simulink model "ALL_JP360_DBW_V6_5_1103"  (R2022a)
settings: Solver=FixedStepAuto  StartTime=0.0  StopTime=inf  FixedStep=0.01  RelTol=1e-3  EnableMultiTasking=on
model workspace (MAT data in the model file):
  g = 9.8
undefined symbols (not defined in the file or in its folder): canChannel, delta_v_p, IPM_Line_C0, IPM_Line_C1, IPM_Line_C2, IPM_Line_C3, M, M_p, MRR_ObjDistX, MRR_ObjDistY, MRR_ObjFusionCamID, MRR_ObjFusionSig, MRR_ObjID, MRR_ObjRelVelX, MRR_ObjRelVelY, MRR_ObjType, MRR_ObjUpdFlg, none, obj_vaild, untracktime, V, videoinput
libraries: canfdmsglib x230, canfdlib x76, slpidlib x24, simulink x18, dspstat3 x14, ctrlSharedLib x1, simulink_extras x1, imaqlib x1, realtime_pacer_lib x1, dspvision x1, visionsinks x1
(part 4 of 55)

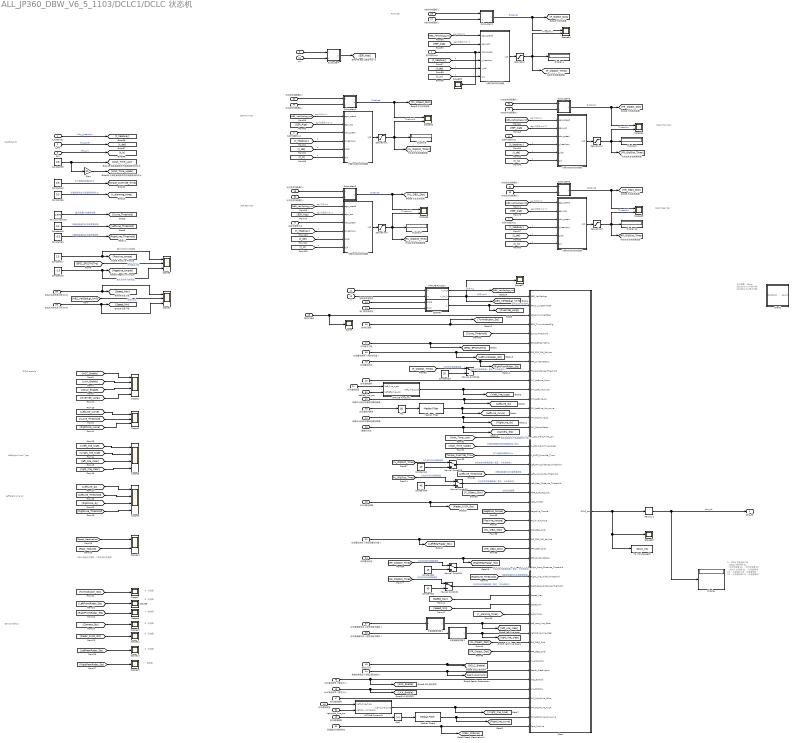
== system ALL_JP360_DBW_V6_5_1103/DCLC1/DCLC状态机 ==
  note: Coefficients
  note: 1表示未越过车道线，2表示越过车道线
  note: 0：无故障
  note: Front Car
  note: Left/Right Line Type
  note: DCLC enable
  note: 运行周期：10ms
      | condition为1开始计数；
      | condition为0停止计数；
  note: ego加速度m/s^2
  note: s
  note: s
  note: s
  note: ego加速度m/s^2
  note: s
  note: 0	：DCLC功能关闭
      | 10	：DCLC功能受限
      | 11	：允许左变道
      | 12	：允许右变道
      | 13	：允许左/右变道
      | 21	：左变道等待
      | 22	：左变道中
      | 23	：左变道回退
      | 24	：左变道结束
      | 31	：右变道等待
      | 32	：右变道中
      | 33	：右变道回退
      | 34	：右变道结束
  note: ego车速m/s
  note: s
  note: s
  note: s
  note: s
  note: ego车速m/s
  note: s
  note: s
  note: ego加速度m/s^2
  note: ego车速m/s
  note: s
  note: ego加速度m/s^2
  note: ego车速m/s
  note: s
  note: s
  note: ego车速m/s
  note: ego加速度m/s^2
  note: s
  note: s
  note: Left/Right Line dy
  note: Left Front Car
  note: Right Front Car
  note: Right Rear Car
  note: Left Rear Car
  note: 0：无故障
  note: 7：有故障
  note: 0：无故障
  note: 0：无故障
  note: 0：无故障
  note: 7：有故障
  note: Sensor Status
  t_headway : Inport
  t_del : Inport  Port=2
  t_lc : Inport  Port=3
  前车速度m/s : Inport  Port=4
  左前车速度m/s : Inport  Port=5
  右前车速度m/s : Inport  Port=6
  右后车速度m/s : Inport  Port=7
  左后车速度m/s : Inport  Port=8
  ax : Inport  Port=9
  ay : Inport  Port=10
  vx : Inport  Port=11
  vy : Inport  Port=12
  刹车信号有效性 : Inport  Port=13
  油门信号有效性 : Inport  Port=14
  转向灯请求 : Inport  Port=15
  转向灯故障 : Inport  Port=16
  方向盘手力矩 : Inport  Port=17
  左前雷达故障（用右前代替） : Inport  Port=18
  右前雷达状态 : Inport  Port=19
  左车道线颜色 : Inport  Port=20
  左车道线类型 : Inport  Port=21
  后轴中心到左车道线的横向距离 : Inport  Port=22
  左车道线的曲率 : Inport  Port=23
  后轴中心到右车道线的横向距离 : Inport  Port=24
  摄像头状态 : Inport  Port=25
  与前车的距离的x : Inport  Port=26
  与前车的距离的y : Inport  Port=27
  1V1R雷达故障 : Inport  Port=28
  与左后车的距离的x : Inport  Port=29
  与左后车的距离的y : Inport  Port=30
  左后雷达失效（用右后雷达代替） : Inport  Port=31
  与右后车的距离的x : Inport  Port=32
  与右后车的距离的y : Inport  Port=33
  右后雷达状态 : Inport  Port=34
  DCLC失效车速上限/km/h : Inport  Port=35
  DCLC失效车速下限/km/h : Inport  Port=36
  左车道清晰状态（信号名暂不确定） : Inport  Port=37
  右车道清晰状态（信号名暂不确定） : Inport  Port=38
  与左前车的距离的x : Inport  Port=39
  与左前车的距离的y : Inport  Port=40
  与右前车的距离的x : Inport  Port=41
  与右前车的距离的y : Inport  Port=42
  DCLC开关 : Inport  Port=43
  换道结束标志（DCLC算法给出） : Inport  Port=44
  ACC激活信号（暂定为1） : Inport  Port=45
  LKA激活信号（暂定为1） : Inport  Port=46
  右车道线颜色 : Inport  Port=47
  右车道线类型 : Inport  Port=48
  右车道线曲率 : Inport  Port=49
  变道越过车道线标志 : Inport  Port=50
  leftleft_line_pro : Inport  Port=51
  rightright_line_pro : Inport  Port=52
  Abs : Abs  SaturateOnIntegerOverflow=off
  Abs1 : Abs  SaturateOnIntegerOverflow=off
  Chart : Stateflow chart  TreatAsAtomicUnit=on
  Chart1 : Stateflow chart  TreatAsAtomicUnit=on
  Constant16 : Constant  Value=-1.5  OutDataTypeStr=single
  Constant17 : Constant  Value=1.5  OutDataTypeStr=single
  Constant23 : Constant  Value=20  OutDataTypeStr=single
  Constant38 : Constant  Value=0.5  OutDataTypeStr=single
  Constant40 : Constant  Value=0.5
  Constant{44,46,60,62} (4 alike) : Constant  Value=45  OutDataTypeStr=single
  Constant45 : Constant  Value=0.5  OutDataTypeStr=single
  Constant61 : Constant  Value=-0.5  OutDataTypeStr=single
  Constant66 : Constant  Value=0.5  OutDataTypeStr=single
  Display{,1,5..6,9..10} (6 alike) : Display
  Gain : Gain  Gain=20  ParamDataTypeStr=single  OutDataTypeStr=single
  MATLAB Function : MATLAB Function  TreatAsAtomicUnit=on
  MATLAB Function2 : MATLAB Function  TreatAsAtomicUnit=on
  MATLAB Function3 : MATLAB Function  TreatAsAtomicUnit=on
  Manual Switch{26,28..31} (5 alike) : ManualSwitch
  Median Filter : dspstat3/Median Filter  WindowLength=5  SimulateUsing=Interpreted execution
      settings: SourceProductBaseCode=DS
  Median Filter1 : dspstat3/Median Filter  WindowLength=5  SimulateUsing=Interpreted execution
      settings: SourceProductBaseCode=DS
  Memory1 : Memory
  Saturation{,1..4} (5 alike) : Saturate  UpperLimit=100  LowerLimit=-100
  Scope{,7..13,53,62,67} (11 alike) : Scope
  Scope1 : Scope  NumInputPorts=3
  Scope{14,54,63..66} (6 alike) : Scope  NumInputPorts=2
  Scope2 : Scope  NumInputPorts=4
  Scope3 : Scope  NumInputPorts=3
  Scope4 : Scope  NumInputPorts=3
  Scope5 : Scope  NumInputPorts=4
  Scope6 : Scope  NumInputPorts=4
  Subsystem : Subsystem
  Subsystem1 : Subsystem
  Subsystem2 : Subsystem
  Subsystem3 : Subsystem
  Subsystem4 : Subsystem
  Subsystem5 : Subsystem
  To Workspace13 : ToWorkspace  VariableName=DCLC_sts  SaveFormat=Timeseries  SampleTime=-1
  max_curve_thres : Constant  Value=1/500
  计算与前车安全距离 : MATLAB Function  TreatAsAtomicUnit=on
  计算与右前车安全距离 : MATLAB Function  TreatAsAtomicUnit=on
  计算与右后车安全距离 : MATLAB Function  TreatAsAtomicUnit=on
  计算与左前车安全距离 : MATLAB Function  TreatAsAtomicUnit=on
  计算与左后车安全距离 : MATLAB Function  TreatAsAtomicUnit=on
  超控判断 : MATLAB Function  TreatAsAtomicUnit=on
  车道清晰度判断1 : MATLAB Function  TreatAsAtomicUnit=on
  车道清晰度判断2 : MATLAB Function  TreatAsAtomicUnit=on
  dclc_sts : Outport
  wires:
  [ESP_Algt] -> 计算与右前车安全距离/2(ego_acc)
  Saturation2/1 -> Scope64/2, [FR_ObjDist_Thres], Display6/1  "Threshold"
  [t_headway] -> 计算与左前车安全距离/4(t_headway)
  [FL_ObjDist_Thres] -> Manual Switch28/1  "与左前车安全距离阈值"
  [ESP_Algt] -> 计算与右后车安全距离/2(ego_acc)
  Constant17/1 -> Scope3/1, [Positive_torque]  "最大正向手力矩阈值"
  [ABS_VehSpdLgt_ms] -> 计算与右后车安全距离/1(ego_speed)
  MATLAB Function/1(v_m_s) -> [ABS_VehSpdLgt_ms]  "车速m/s"
  [ABS_VehSpdLgt_ms] -> 计算与右前车安全距离/1(ego_speed)
  Constant62/1 -> Manual Switch31/2
  前车速度m/s/1 -> Scope53/1, 计算与前车安全距离/3(obs_speed)
  [ESP_Algt] -> 计算与前车安全距离/2(ego_acc)
  右后雷达状态/1 -> [RightRearRadar_Sts], Chart/29(RRR_SystemStatus)
  Constant44/1 -> Manual Switch28/2
  t_del/1 -> [t_del]  "obs_t_del"
  计算与前车安全距离/1(L2S) -> Saturation/1
  [ESP_Algt] -> 计算与左前车安全距离/2(ego_acc)
  max_curve_thres/1 -> [Curve_Threshold]  "最大能通行的曲率阈值"
  [t_headway] -> 计算与右前车安全距离/4(t_headway)
  [t_lc] -> 计算与左后车安全距离/6(t_lc)
  [t_del] -> 计算与左后车安全距离/5(t_del)
  [ABS_VehSpdLgt_ms] -> 计算与前车安全距离/1(ego_speed)
  Manual Switch31/1 -> Chart/32(Right_Rear_Distance_Threshold)  "与右后车的距离阈值（暂定，与车速有关）"
  与右前车的距离的y/1 -> Subsystem5/2(y)
  [t_lc] -> 计算与右前车安全距离/6(t_lc)
  [t_lc] -> 计算与右后车安全距离/6(t_lc)
  [t_headway] -> 计算与左后车安全距离/4(t_headway)
  计算与右前车安全距离/1(L2S) -> Saturation2/1
  [t_del] -> 计算与右前车安全距离/5(t_del)
  [t_del] -> 计算与前车安全距离/5(t_del)
  Subsystem1/1(u) -> Scope54/1, [F_Object_Dist]  "Distance"
  [FR_ObjDist_Thres] -> Manual Switch30/1  "与右前车安全距离阈值"
  [ABS_VehSpdLgt_ms] -> 计算与左后车安全距离/1(ego_speed)
  Manual Switch30/1 -> Chart/30(Right_Front_Distance_Threshold)  "与右前车的距离阈值（暂定，与车速有关）"
  t_lc/1 -> [t_lc]  "obs_t_lc"
  [t_headway] -> 计算与右后车安全距离/4(t_headway)
  左后车速度m/s/1 -> 计算与左后车安全距离/3(obs_speed)
  [ESP_Algt] -> 计算与左后车安全距离/2(ego_acc)
  [t_lc] -> 计算与前车安全距离/6(t_lc)
  Constant45/1 -> [LeftLine_Threshold]  "判断能换道的左车道宽度阈值"
  [t_del] -> 计算与左前车安全距离/5(t_del)
  左前雷达故障（用右前代替）/1 -> [LeftFrontRadar_Sts], Chart/7(FLR_SRR_Obj_Failure)
  计算与左后车安全距离/1(L2S) -> Saturation4/1
  Constant46/1 -> Manual Switch29/2
  [ABS_VehSpdLgt_ms] -> 计算与左前车安全距离/1(ego_speed)
  与右后车的距离的y/1 -> Subsystem3/2(y)
  Saturation4/1 -> Scope66/2, [RL_ObjDist_Thres], Display9/1  "Threshold"
  DCLC失效车速上限/km/h/1 -> Scope1/1, [Speed_Max]
  Constant16/1 -> Scope3/3, [Negative_torque]  "最大反向手力矩阈值"
  [t_lc] -> 计算与左前车安全距离/6(t_lc)
  [RL_ObjDist_Thres] -> Manual Switch29/1  "与左后车安全距离阈值"
  Subsystem/1(u) -> [ESP_Algt]
  Constant61/1 -> [RightLine_Threshold]  "判断能换道的右车道宽度阈值"
  Constant60/1 -> Manual Switch30/2
  Saturation/1 -> Scope54/2, Display1/1, [F_ObjDist_Thres]  "Threshold"
  [F_ObjDist_Thres] -> Manual Switch26/1  "与前车安全距离阈值"
  [t_headway] -> 计算与前车安全距离/4(t_headway)
  [t_del] -> 计算与右后车安全距离/5(t_del)
  DCLC失效车速下限/km/h/1 -> Scope1/3, [Speed_Min]
  Manual Switch29/1 -> Chart/21(Left_Rear_Distance_Threshold)  "与左后车的距离阈值（暂定，与车速有关）"
  Saturation3/1 -> Scope65/2, [RR_ObjDist_Thres], Display10/1  "Threshold"
  Subsystem2/1(u) -> Scope66/1, [RL_OBJ1_Dist]  "Distance"
  Manual Switch28/1 -> Chart/19(Left_Front_Distance_Threshold)  "与左前车的距离阈值（暂定，与车速有关）"
  与左后车的距离的x/1 -> Subsystem2/1(x)
  Subsystem4/1(u) -> Scope63/1, [FL_Object_Dist]  "Distance"
  转向灯请求/1 -> Chart/3(ADU1_TurnLightReq), Scope/1
  与右后车的距离的x/1 -> Subsystem3/1(x)
  Manual Switch26/1 -> Chart/9(Front_Distance_Threshold)  "与前车的距离阈值（暂定，与车速有关）"
  Saturation1/1 -> Scope63/2, [FL_ObjDist_Thres], Display5/1  "Threshold"
  [RR_ObjDist_Thres] -> Manual Switch31/1  "与右后车安全距离阈值"
  Subsystem5/1(u) -> Scope64/1, [FR_Object_Dist]  "Distance"
  t_headway/1 -> [t_headway]  "obs_t_headway"
  MATLAB Function/2(v_km_h) -> [ABS_VehSpdLgt_kmh], Scope67/1, Chart/1(ABS_VehSpdLgt)  "车速 km/h"
  Constant23/1 -> Manual Switch26/2
  1V1R雷达故障/1 -> [Radar_1V1R_Sts], Chart/23(MRR_HWFail)
  计算与右后车安全距离/1(L2S) -> Saturation3/1
  超控判断/1(u) -> [Override_Longi], Chart/2(ADU1_LongCtrlMode)  "纵向override信号"
  Chart/1(DCLC_sts) -> Memory1/1, To Workspace13/1, Scope62/1
  计算与左前车安全距离/1(L2S) -> Saturation1/1
  Subsystem3/1(u) -> Scope65/1, [RR_OBJ1_Dist]  "Distance"
  车道清晰度判断2/1(y) -> [right_line_clear], Chart/37(right_lane_line_clear)
  车道清晰度判断1/1(y) -> [left_line_clear], Chart/36(left_lane_line_clear)
  后轴中心到右车道线的横向距离/1 -> [RightLine_dy], Chart/14(IPM_RightLine_dy)
  DCLC开关/1 -> [DCLC_Enable], Chart/40(IVI_DCLC_ON)
  方向盘手力矩/1 -> [EPS2_EPS1TASTrq], Chart/6(EPS2_EPS1TASTrq)
  右前雷达状态/1 -> [RightFrontRadar_Sts], Chart/8(FRR_SystemStatus)
  后轴中心到左车道线的横向距离/1 -> [LeftLine_dy], Chart/12(IPM_LeftLine_dy)
  左后雷达失效（用右后雷达代替）/1 -> Chart/27(RLR_SRR_Obj_Failure), [LeftRearRadar_Sts]
  与前车的距离的y/1 -> Subsystem1/2(y)
  左车道清晰状态（信号名暂不确定）/1 -> 车道清晰度判断1/1(u)
  左前车速度m/s/1 -> 计算与左前车安全距离/3(obs_speed)
  转向灯故障/1 -> [TurnIndicator_Sts], Chart/4(BCM_TurnIndicatorDig)
  摄像头状态/1 -> [Camera_Sts], Chart/15(IPM_SensorState)
  右前车速度m/s/1 -> 计算与右前车安全距离/3(obs_speed)
  vx/1 -> MATLAB Function/1(vx)
  左车道线的曲率/1 -> Abs/1
  ax/1 -> Subsystem/1(x)
  ay/1 -> Subsystem/2(y)
  右后车速度m/s/1 -> 计算与右后车安全距离/3(obs_speed)
  换道结束标志（DCLC算法给出）/1 -> [Reach_Destination], Chart/41(Reach_Destination)
  与前车的距离的x/1 -> Subsystem1/1(x)
  与左后车的距离的y/1 -> Subsystem2/2(y)
  油门信号有效性/1 -> 超控判断/2(throt)
  Memory1/1 -> dclc_sts/1, Display/1  "dclc_sts"
  与左前车的距离的y/1 -> Subsystem4/2(y)
  与右前车的距离的x/1 -> Subsystem5/1(x)
  与左前车的距离的x/1 -> Subsystem4/1(x)
  ACC激活信号（暂定为1）/1 -> [ACC_Enable], Chart/42(ACC_Enable)
  右车道清晰状态（信号名暂不确定）/1 -> 车道清晰度判断2/1(u)
  刹车信号有效性/1 -> 超控判断/1(brake)
  LKA激活信号（暂定为1）/1 -> [LKA_Enable], Chart/43(LKA_Enable)
  vy/1 -> MATLAB Function/2(vy)
  右车道线颜色/1 -> Chart/44(IPM_RightLine_Color)
  右车道线曲率/1 -> Abs1/1
  左车道线颜色/1 -> Chart/10(IPM_LeftLine_Color)
  变道越过车道线标志/1 -> [Pass_MidLine], Chart/47(Pass_Midline)
  左车道线类型/1 -> MATLAB Function2/1(left_line_type)
  leftleft_line_pro/1 -> MATLAB Function2/2(leftleft_line_pro)
  MATLAB Function2/1(vleft_line_type) -> [Vleft_line_type], Chart/11(IPM_LeftLine_Type)
  右车道线类型/1 -> MATLAB Function3/1(right_line_type)
  rightright_line_pro/1 -> MATLAB Function3/2(rightright_line_pro)
  MATLAB Function3/1(vright_line_type) -> [Vright_line_type], Chart/45(IPM_RightLine_Type)
  [ABS_VehSpdLgt_kmh] -> Scope1/2  "车速km/h"
  [ACC_Enable] -> Scope2/1
  [LKA_Enable] -> Scope2/2
  [DCLC_Enable] -> Scope2/3
  [EPS2_EPS1TASTrq] -> Scope3/2  "方向盘手力矩"
  [LeftLine_curve] -> Scope4/1
  [Curve_Threshold] -> Scope4/2
  [RightLine_curve] -> Scope4/3
  [Override_Longi] -> Scope2/4
  [Vleft_line_type] -> Scope5/1
  [Vright_line_type] -> Scope5/2
  [left_line_clear] -> Scope5/3
  [right_line_clear] -> Scope5/4
  [LeftLine_dy] -> Scope6/1
  [LeftLine_Threshold] -> Scope6/2
  [RightLine_dy] -> Scope6/3
  [RightLine_Threshold] -> Scope6/4
  [TurnIndicator_Sts] -> Scope7/1
  [LeftFrontRadar_Sts] -> Scope8/1
  [RightFrontRadar_Sts] -> Scope9/1
  [Camera_Sts] -> Scope10/1
  [Radar_1V1R_Sts] -> Scope11/1
  [LeftRearRadar_Sts] -> Scope12/1
  [RightRearRadar_Sts] -> Scope13/1
  [Reach_Destination] -> Scope14/1
  [Pass_MidLine] -> Scope14/2
  Abs/1 -> Median Filter/1
  Abs1/1 -> Median Filter1/1
  Median Filter/1 -> [LeftLine_curve], Chart/13(IPM_LeftLine_hor_curve)
  Median Filter1/1 -> [RightLine_curve], Chart/46(IPM_RightLine_hor_curve)
  [Curve_Threshold] -> Chart/5(Curve_Threshold)
  Constant38/1 -> Gain/1, [Wait_Time_Low]
  [Wait_Time_Low] -> Chart/16(K_LCD_Wait_Time_Low)  "满足换道条件开始换道时间下限/s"
  [Wait_Time_Upper] -> Chart/17(K_LCD_Wait_Time_Upper)  "不满足换道条件取消换道时间上限/s"
  Gain/1 -> [Wait_Time_Upper]
  Constant40/1 -> [Torque_Override_Time]  "手力矩超时阈值时间/s"
  [Torque_Override_Time] -> Chart/18(K_SACC_Override_Time)  "手力矩超时阈值时间/s"
  [LeftLine_Threshold] -> Chart/20(Left_Line_Width_Threshold)  "判断能换道的左车道宽度阈值"
  [F_Object_Dist] -> Chart/22(MRR_F_Object_dist)  "与前车的距离"
  [Negative_torque] -> Chart/24(Negative_Torque)
  [Positive_torque] -> Chart/25(Positive_Torque)
  [RL_OBJ1_Dist] -> Chart/26(RLR_OBJ1_Dist)
  [RR_OBJ1_Dist] -> Chart/28(RRR_OBJ1_Dist)
  [RightLine_Threshold] -> Chart/31(Right_Line_Width_Threshold)  "判断能换道的右车道宽度阈值"
  [Speed_Max] -> Chart/33(Speed_Max)
  [Speed_Min] -> Chart/34(Speed_Min)
  Constant66/1 -> [t_planning_thres]  "变道结束到允许变道等待时间/s"
  [t_planning_thres] -> Chart/35(t_planning)
  [FL_Object_Dist] -> Chart/38(FLR_OBJ1_Dist)
  [FR_Object_Dist] -> Chart/39(FRR_OBJ1_Dist)

== system ALL_JP360_DBW_V6_5_1103/DCLC1/LQR ==
  vx : Inport
  xrr : Inport  Port=2
  yrr : Inport  Port=3
  thetar : Inport  Port=4
  kappar : Inport  Port=5
  Add : Sum
  Constant : Constant  Value=0.26
  Constant1 : Constant  OutDataTypeStr=double
  Constant113 : Constant  Commented=on  Value=1.276  OutDataTypeStr=single
  Constant114 : Constant  Commented=on  Value=1.589  OutDataTypeStr=single
  Constant115 : Constant  Commented=on  Value=1830  OutDataTypeStr=single
  Constant116 : Constant  Commented=on  Value=-155493.663  OutDataTypeStr=single
  Constant117 : Constant  Commented=on  Value=-155493.663  OutDataTypeStr=single
  Constant2 : Constant  Value=0.01  OutDataTypeStr=double
  Constant3 : Constant  Value=0  OutDataTypeStr=double
  Constant4 : Constant  Value=0  OutDataTypeStr=double
  Constant5 : Constant  Value=0.3  OutDataTypeStr=single
  Gain11 : Gain  Gain=180/pi  ParamDataTypeStr=single  OutDataTypeStr=single
  Gain7 : Gain  Gain=15.9  ParamDataTypeStr=single  OutDataTypeStr=single
  LQR_offline : MATLAB Function  TreatAsAtomicUnit=on
  MATLAB Function1 : MATLAB Function  TreatAsAtomicUnit=on
  Scope4 : Scope  Commented=on
  Sum5 : Sum  Inputs=|++
  err kappa calculate module : MATLAB Function  TreatAsAtomicUnit=on
  forward_angle1 : MATLAB Function  Commented=on  TreatAsAtomicUnit=on
  steering_angle : Outport
  wires:
  err kappa calculate module/1(kr) -> forward_angle1/8(kr)
  vx/1 -> forward_angle1/6(vx), LQR_offline/5(vx), err kappa calculate module/1(vx)
  yrr/1 -> LQR_offline/7(yr), err kappa calculate module/3(yr)
  thetar/1 -> err kappa calculate module/4(thetar)
  Constant2/1 -> LQR_offline/1(k1)
  Constant113/1 -> forward_angle1/1(a)
  Sum5/1 -> Gain11/1
  Constant116/1 -> forward_angle1/4(cf)
  err kappa calculate module/2(err) -> MATLAB Function1/2(err)  "err"
  Constant115/1 -> forward_angle1/3(m)
  forward_angle1/1(forward_angle) -> Scope4/1
  MATLAB Function1/1(lqr_angle) -> Sum5/2
  LQR_offline/1(k) -> MATLAB Function1/1(k), forward_angle1/7(k)
  Constant114/1 -> forward_angle1/2(b)
  Constant117/1 -> forward_angle1/5(cr)
  Constant3/1 -> LQR_offline/2(k2)
  Gain11/1 -> Gain7/1
  kappar/1 -> LQR_offline/6(kappa), err kappa calculate module/5(kappar)
  Constant/1 -> LQR_offline/4(k4)
  Constant1/1 -> LQR_offline/3(k3)
  Constant4/1 -> Sum5/1
  xrr/1 -> err kappa calculate module/2(xr)
  Constant5/1 -> Add/2
  Gain7/1 -> Add/1
  Add/1 -> steering_angle/1

== system ALL_JP360_DBW_V6_5_1103/DCLC1/steering_angle_to_torque ==
  desire_steering_angle : Inport
  acture_steering_angle : Inport  Port=2
  vx km/h : Inport  Port=3
  vy km/h : Inport  Port=4
  2-D Lookup Table : Lookup_n-D  DataSpecification=Lookup table object  LookupTableObject=lat_calibration3  BreakpointsForDimension1=[1:3]  BreakpointsForDimension2=[1:3]  InternalRulePriority=Speed  RndMeth=Simplest
      settings: InputPortMap=u0,u1
  Add : Sum
  Gain : Gain  Gain=0.9
  Product : Product
  Product1 : Product
  Sqrt : Sqrt
  torque : Outport
  wires:
  vx km/h/1 -> Product/2, Product/1
  vy km/h/1 -> Product1/2, Product1/1
  Product/1 -> Add/1
  Product1/1 -> Add/2
  Add/1 -> Sqrt/1
  Sqrt/1 -> 2-D Lookup Table/1  "speed km/h"
  desire_steering_angle/1 -> 2-D Lookup Table/2
  2-D Lookup Table/1 -> Gain/1
  Gain/1 -> torque/1

== system ALL_JP360_DBW_V6_5_1103/LKA_Control/LKA_Cal ==
  note: DegToRad
  Ct : Inport  OutDataTypeStr=single
  LKA_status : Inport  Port=2
  SAS_SteerWheelAngle : Inport  Port=3
  ABS_Vhlspd : Inport  Port=4
  ErrorCal : Subsystem
  Gain1 : Gain  Gain=pi/180  ParamDataTypeStr=single  OutDataTypeStr=single
  LKAControlerl : Subsystem
  LKAReq_angle : Outport
  err_now : Outport  Port=2
  wires:
  Ct/1 -> ErrorCal/2(Ct)
  ErrorCal/1(LatErr) -> LKAControlerl/2(LatErr)
  ABS_Vhlspd/1 -> LKAControlerl/1(ABS_VehSpd), ErrorCal/1(ABS_Vhlspd)
  LKAControlerl/1(SteeringAngleCommand) -> LKAReq_angle/1
  ErrorCal/2(err_now) -> LKAControlerl/3(err_now), err_now/1
  ErrorCal/3(thetar) -> LKAControlerl/4(Line_theta)
  Gain1/1 -> ErrorCal/3(SAS_SteerWheelAngle1)
  LKA_status/1 -> LKAControlerl/6(LKA_status)
  SAS_SteerWheelAngle/1 -> Gain1/1, LKAControlerl/5(steer_angle)

== system ALL_JP360_DBW_V6_5_1103/LKA_Control/Lane_Status ==
  LRC : Inport
  IPM_Line01_Existence_Probability : Inport  Port=2
  IPM_Line02_Existence_Probability : Inport  Port=3
  Demux : Demux  Outputs=8
  Lane_analyse : MATLAB Function  TreatAsAtomicUnit=on
  To Workspace1 : ToWorkspace  VariableName=Cl0  SaveFormat=Structure With Time  SampleTime=-1
  To Workspace2 : ToWorkspace  VariableName=Cr0  SaveFormat=Structure With Time  SampleTime=-1
  Ct : Outport
  lane_status : Outport  Port=2  OutDataTypeStr=int8
  ang : Outport  Port=3
  C2 : Outport  Port=4
  wires:
  Demux/1 -> To Workspace1/1, Lane_analyse/1(Cl0)
  Demux/5 -> To Workspace2/1, Lane_analyse/5(Cr0)
  Lane_analyse/2(lane_status) -> lane_status/1
  LRC/1 -> Demux/1
  Lane_analyse/1(Ct) -> Ct/1
  IPM_Line01_Existence_Probability/1 -> Lane_analyse/9(L_p)
  IPM_Line02_Existence_Probability/1 -> Lane_analyse/10(R_p)
  Demux/2 -> Lane_analyse/2(Cl1)
  Demux/3 -> Lane_analyse/3(Cl2)
  Demux/4 -> Lane_analyse/4(Cl3)
  Demux/6 -> Lane_analyse/6(Cr1)
  Demux/7 -> Lane_analyse/7(Cr2)
  Demux/8 -> Lane_analyse/8(Cr3)
  Lane_analyse/3(ang) -> ang/1
  Lane_analyse/4(C2) -> C2/1

== system ALL_JP360_DBW_V6_5_1103/MsgFromCAN/ADCU_data ==
  CAN FD Receive1 : canfdlib/CAN FD Receive  BlockHandle=78235.0004  Device=Vector VN1640A 1 (Channel 3)  ObjConstructor=canChannel('Vector', 'VN1640A 1', 3, 'ProtocolMode', 'CAN FD')  EnableStandardIDsFilter=off  StdIDsCombo=Allow only  StandardIDs=545  EnableExtendedIDsFilter=off  ExtIDsCombo=Allow all  ExtendedIDs=0  SampleTime=0.01  MsgsPerTimestep=all  InternalFilterUpdateStatus=on  BusOutput=on
      settings: SourceProductBaseCode=VN
  CAN FD Receive10 : canfdlib/CAN FD Receive  BlockHandle=78239.0004  Device=Vector VN1640A 1 (Channel 3)  ObjConstructor=canChannel('Vector', 'VN1640A 1', 3, 'ProtocolMode', 'CAN FD')  EnableStandardIDsFilter=off  StdIDsCombo=Allow only  StandardIDs=263  EnableExtendedIDsFilter=off  ExtIDsCombo=Allow all  ExtendedIDs=0  SampleTime=0.01  MsgsPerTimestep=all  InternalFilterUpdateStatus=on  BusOutput=on
      settings: SourceProductBaseCode=VN
  CAN FD Receive11 : canfdlib/CAN FD Receive  BlockHandle=78242.0004  Device=Vector VN1640A 1 (Channel 3)  ObjConstructor=canChannel('Vector', 'VN1640A 1', 3, 'ProtocolMode', 'CAN FD')  EnableStandardIDsFilter=off  StdIDsCombo=Allow only  StandardIDs=1296  EnableExtendedIDsFilter=off  ExtIDsCombo=Allow all  ExtendedIDs=0  SampleTime=0.01  MsgsPerTimestep=all  InternalFilterUpdateStatus=on  BusOutput=on
      settings: SourceProductBaseCode=VN
  CAN FD Receive12 : canfdlib/CAN FD Receive  BlockHandle=78245.0004  Device=Vector VN1640A 1 (Channel 3)  ObjConstructor=canChannel('Vector', 'VN1640A 1', 3, 'ProtocolMode', 'CAN FD')  EnableStandardIDsFilter=off  StdIDsCombo=Allow only  StandardIDs=848  EnableExtendedIDsFilter=off  ExtIDsCombo=Allow all  ExtendedIDs=0  SampleTime=0.01  MsgsPerTimestep=all  InternalFilterUpdateStatus=on  BusOutput=on
      settings: SourceProductBaseCode=VN
  CAN FD Receive13 : canfdlib/CAN FD Receive  BlockHandle=78248.0004  Device=Vector VN1640A 1 (Channel 3)  ObjConstructor=canChannel('Vector', 'VN1640A 1', 3, 'ProtocolMode', 'CAN FD')  EnableStandardIDsFilter=off  StdIDsCombo=Allow only  StandardIDs=291  EnableExtendedIDsFilter=off  ExtIDsCombo=Allow all  ExtendedIDs=0  SampleTime=0.01  MsgsPerTimestep=all  InternalFilterUpdateStatus=on  BusOutput=on
      settings: SourceProductBaseCode=VN
  CAN FD Receive14 : canfdlib/CAN FD Receive  BlockHandle=78251.0004  Device=Vector VN1640A 1 (Channel 3)  ObjConstructor=canChannel('Vector', 'VN1640A 1', 3, 'ProtocolMode', 'CAN FD')  EnableStandardIDsFilter=off  StdIDsCombo=Allow only  StandardIDs=373  EnableExtendedIDsFilter=off  ExtIDsCombo=Allow all  ExtendedIDs=0  SampleTime=0.01  MsgsPerTimestep=all  InternalFilterUpdateStatus=on  BusOutput=on
      settings: SourceProductBaseCode=VN
  CAN FD Receive15 : canfdlib/CAN FD Receive  BlockHandle=78254.0004  Device=Vector VN1640A 1 (Channel 3)  ObjConstructor=canChannel('Vector', 'VN1640A 1', 3, 'ProtocolMode', 'CAN FD')  EnableStandardIDsFilter=off  StdIDsCombo=Allow only  StandardIDs=794  EnableExtendedIDsFilter=off  ExtIDsCombo=Allow all  ExtendedIDs=0  SampleTime=0.01  MsgsPerTimestep=all  InternalFilterUpdateStatus=on  BusOutput=on
      settings: SourceProductBaseCode=VN
  CAN FD Receive16 : canfdlib/CAN FD Receive  BlockHandle=78257.0004  Device=Vector VN1640A 1 (Channel 3)  ObjConstructor=canChannel('Vector', 'VN1640A 1', 3, 'ProtocolMode', 'CAN FD')  EnableStandardIDsFilter=off  StdIDsCombo=Allow only  StandardIDs=795  EnableExtendedIDsFilter=off  ExtIDsCombo=Allow all  ExtendedIDs=0  SampleTime=0.01  MsgsPerTimestep=all  InternalFilterUpdateStatus=on  BusOutput=on
      settings: SourceProductBaseCode=VN
  CAN FD Receive17 : canfdlib/CAN FD Receive  BlockHandle=78260.0004  Device=Vector VN1640A 1 (Channel 3)  ObjConstructor=canChannel('Vector', 'VN1640A 1', 3, 'ProtocolMode', 'CAN FD')  EnableStandardIDsFilter=off  StdIDsCombo=Allow only  StandardIDs=257  EnableExtendedIDsFilter=off  ExtIDsCombo=Allow all  ExtendedIDs=0  SampleTime=0.01  MsgsPerTimestep=all  InternalFilterUpdateStatus=on  BusOutput=on
      settings: SourceProductBaseCode=VN
  CAN FD Receive2 : canfdlib/CAN FD Receive  BlockHandle=78263.0004  Device=Vector VN1640A 1 (Channel 3)  ObjConstructor=canChannel('Vector', 'VN1640A 1', 3, 'ProtocolMode', 'CAN FD')  EnableStandardIDsFilter=off  StdIDsCombo=Allow only  StandardIDs=374  EnableExtendedIDsFilter=off  ExtIDsCombo=Allow all  ExtendedIDs=0  SampleTime=0.01  MsgsPerTimestep=all  InternalFilterUpdateStatus=on  BusOutput=on
      settings: SourceProductBaseCode=VN
  CAN FD Receive3 : canfdlib/CAN FD Receive  BlockHandle=78266.0004  Device=Vector VN1640A 1 (Channel 3)  ObjConstructor=canChannel('Vector', 'VN1640A 1', 3, 'ProtocolMode', 'CAN FD')  EnableStandardIDsFilter=off  StdIDsCombo=Allow only  StandardIDs=578  EnableExtendedIDsFilter=off  ExtIDsCombo=Allow all  ExtendedIDs=0  SampleTime=0.01  MsgsPerTimestep=all  InternalFilterUpdateStatus=on  BusOutput=on
      settings: SourceProductBaseCode=VN
  CAN FD Receive4 : canfdlib/CAN FD Receive  BlockHandle=78269.0004  Device=Vector VN1640A 1 (Channel 3)  ObjConstructor=canChannel('Vector', 'VN1640A 1', 3, 'ProtocolMode', 'CAN FD')  EnableStandardIDsFilter=off  StdIDsCombo=Allow only  StandardIDs=565  EnableExtendedIDsFilter=off  ExtIDsCombo=Allow all  ExtendedIDs=0  SampleTime=0.01  MsgsPerTimestep=all  InternalFilterUpdateStatus=on  BusOutput=on
      settings: SourceProductBaseCode=VN
  CAN FD Receive5 : canfdlib/CAN FD Receive  BlockHandle=78272.0004  Device=Vector VN1640A 1 (Channel 3)  ObjConstructor=canChannel('Vector', 'VN1640A 1', 3, 'ProtocolMode', 'CAN FD')  EnableStandardIDsFilter=off  StdIDsCombo=Allow only  StandardIDs=577  EnableExtendedIDsFilter=off  ExtIDsCombo=Allow all  ExtendedIDs=0  SampleTime=0.01  MsgsPerTimestep=all  InternalFilterUpdateStatus=on  BusOutput=on
      settings: SourceProductBaseCode=VN
  CAN FD Receive6 : canfdlib/CAN FD Receive  BlockHandle=78275.0004  Device=Vector VN1640A 1 (Channel 3)  ObjConstructor=canChannel('Vector', 'VN1640A 1', 3, 'ProtocolMode', 'CAN FD')  EnableStandardIDsFilter=off  StdIDsCombo=Allow only  StandardIDs=579  EnableExtendedIDsFilter=off  ExtIDsCombo=Allow all  ExtendedIDs=0  SampleTime=0.01  MsgsPerTimestep=all  InternalFilterUpdateStatus=on  BusOutput=on
      settings: SourceProductBaseCode=VN
  CAN FD Receive7 : canfdlib/CAN FD Receive  BlockHandle=78278.0004  Device=Vector VN1640A 1 (Channel 3)  ObjConstructor=canChannel('Vector', 'VN1640A 1', 3, 'ProtocolMode', 'CAN FD')  EnableStandardIDsFilter=off  StdIDsCombo=Allow only  StandardIDs=784  EnableExtendedIDsFilter=off  ExtIDsCombo=Allow all  ExtendedIDs=0  SampleTime=0.01  MsgsPerTimestep=all  InternalFilterUpdateStatus=on  BusOutput=on
      settings: SourceProductBaseCode=VN
  CAN FD Receive8 : canfdlib/CAN FD Receive  BlockHandle=78281.0004  Device=Vector VN1640A 1 (Channel 3)  ObjConstructor=canChannel('Vector', 'VN1640A 1', 3, 'ProtocolMode', 'CAN FD')  EnableStandardIDsFilter=off  StdIDsCombo=Allow only  StandardIDs=801  EnableExtendedIDsFilter=off  ExtIDsCombo=Allow all  ExtendedIDs=0  SampleTime=0.01  MsgsPerTimestep=all  InternalFilterUpdateStatus=on  BusOutput=on
      settings: SourceProductBaseCode=VN
  CAN FD Receive9 : canfdlib/CAN FD Receive  BlockHandle=78284.0004  Device=Vector VN1640A 1 (Channel 3)  ObjConstructor=canChannel('Vector', 'VN1640A 1', 3, 'ProtocolMode', 'CAN FD')  EnableStandardIDsFilter=off  StdIDsCombo=Allow only  StandardIDs=273  EnableExtendedIDsFilter=off  ExtIDsCombo=Allow all  ExtendedIDs=0  SampleTime=0.01  MsgsPerTimestep=all  InternalFilterUpdateStatus=on  BusOutput=on
      settings: SourceProductBaseCode=VN
  Terminator{,1..14,24,29} (17 alike) : Terminator
  CCAN_ADCU_ABS_Sts_0x221FromInData : Outport
  CCAN_ADCU_EPS_Advanced_0x176FromInData : Outport  Port=2
  CCAN_ADCU_ESP_AxAy_0x242FromInData : Outport  Port=3
  CCAN_ADCU_ESP_Direction_0x235FromInData : Outport  Port=4
  CCAN_ADCU_ESP_Pressure_0x241FromInData : Outport  Port=5
  CCAN_ADCU_ESP_Status_0x243FromInData : Outport  Port=6
  CCAN_ADCU_GW_BCM_Door_0x310FromInData : Outport  Port=7
  CCAN_ADCU_GW_Body_0x321FromInData : Outport  Port=8
  CCAN_ADCU_GW_EMS_TqWhl_0x111FromInData : Outport  Port=9
  CCAN_ADCU_GW_EMS_WhlTq_0x107FromInData : Outport  Port=10
  CCAN_ADCU_GW_IC_0x510FromInData : Outport  Port=11
  CCAN_ADCU_GW_SRS_0x350FromInData : Outport  Port=12
  CCAN_ADCU_GW_TCU_GearInfo_0x123FromInData : Outport  Port=13
  CCAN_ADCU_SAS_Sensor_0x175FromInData : Outport  Port=14
  CCAN_ADCU_SWM_Body_0x31AFromInData : Outport  Port=15
  CCAN_ADCU_SWM_MRR_0x31BFromInData : Outport  Port=16
  CCAN_ADCU_ABS_Sts_0x221FromInData1 : Outport  Port=17
  wires:
  CAN FD Receive6/1 -> Terminator5/1
  CAN FD Receive5/2 -> CCAN_ADCU_ESP_Pressure_0x241FromInData/1
  CAN FD Receive7/2 -> CCAN_ADCU_GW_BCM_Door_0x310FromInData/1
  CAN FD Receive6/2 -> CCAN_ADCU_ESP_Status_0x243FromInData/1
  CAN FD Receive8/2 -> CCAN_ADCU_GW_Body_0x321FromInData/1
  CAN FD Receive9/2 -> CCAN_ADCU_GW_EMS_TqWhl_0x111FromInData/1
  CAN FD Receive13/1 -> Terminator11/1
  CAN FD Receive15/1 -> Terminator29/1
  CAN FD Receive14/2 -> CCAN_ADCU_SAS_Sensor_0x175FromInData/1
  CAN FD Receive11/1 -> Terminator24/1
  CAN FD Receive12/1 -> Terminator10/1
  CAN FD Receive13/2 -> CCAN_ADCU_GW_TCU_GearInfo_0x123FromInData/1
  CAN FD Receive16/1 -> Terminator13/1
  CAN FD Receive11/2 -> CCAN_ADCU_GW_IC_0x510FromInData/1
  CAN FD Receive12/2 -> CCAN_ADCU_GW_SRS_0x350FromInData/1
  CAN FD Receive15/2 -> CCAN_ADCU_SWM_Body_0x31AFromInData/1
  CAN FD Receive14/1 -> Terminator12/1
  CAN FD Receive16/2 -> CCAN_ADCU_SWM_MRR_0x31BFromInData/1
  CAN FD Receive1/2 -> CCAN_ADCU_ABS_Sts_0x221FromInData/1
  CAN FD Receive4/2 -> CCAN_ADCU_ESP_Direction_0x235FromInData/1
  CAN FD Receive4/1 -> Terminator3/1
  CAN FD Receive2/2 -> CCAN_ADCU_EPS_Advanced_0x176FromInData/1
  CAN FD Receive7/1 -> Terminator6/1
  CAN FD Receive5/1 -> Terminator4/1
  CAN FD Receive3/2 -> CCAN_ADCU_ESP_AxAy_0x242FromInData/1
  CAN FD Receive8/1 -> Terminator7/1
  CAN FD Receive10/2 -> CCAN_ADCU_GW_EMS_WhlTq_0x107FromInData/1
  CAN FD Receive1/1 -> Terminator/1
  CAN FD Receive10/1 -> Terminator9/1
  CAN FD Receive3/1 -> Terminator2/1
  CAN FD Receive2/1 -> Terminator1/1
  CAN FD Receive9/1 -> Terminator8/1
  CAN FD Receive17/1 -> Terminator14/1
  CAN FD Receive17/2 -> CCAN_ADCU_ABS_Sts_0x221FromInData1/1

== system ALL_JP360_DBW_V6_5_1103/MsgFromCAN/CCAN_ADCU_MsgFromCAN ==
  CCAN_ADCU_ABS_Sts_0x221FromInData : Inport  OutDataTypeStr=Bus:CAN_FD_MESSAGE_BUS
  CCAN_ADCU_BSD_0x275FromInData : Inport  Port=2  OutDataTypeStr=Bus:CAN_FD_MESSAGE_BUS
  CCAN_ADCU_EPS_Advanced_0x176FromInData : Inport  Port=3  OutDataTypeStr=Bus:CAN_FD_MESSAGE_BUS
  CCAN_ADCU_ESP_Advanced_0x234FromInData : Inport  Port=4  OutDataTypeStr=Bus:CAN_FD_MESSAGE_BUS
  CCAN_ADCU_ESP_AxAy_0x242FromInData : Inport  Port=5  OutDataTypeStr=Bus:CAN_FD_MESSAGE_BUS
  CCAN_ADCU_ESP_Direction_0x235FromInData : Inport  Port=6  OutDataTypeStr=Bus:CAN_FD_MESSAGE_BUS
  CCAN_ADCU_ESP_Pressure_0x241FromInData : Inport  Port=7  OutDataTypeStr=Bus:CAN_FD_MESSAGE_BUS
  CCAN_ADCU_ESP_RAW_0x212FromInData : Inport  Port=8  OutDataTypeStr=Bus:CAN_FD_MESSAGE_BUS
  CCAN_ADCU_ESP_Status_0x243FromInData : Inport  Port=9  OutDataTypeStr=Bus:CAN_FD_MESSAGE_BUS
  CCAN_ADCU_GW_AWD_0x251FromInData : Inport  Port=10  OutDataTypeStr=Bus:CAN_FD_MESSAGE_BUS
  CCAN_ADCU_GW_BCM_Door_0x310FromInData : Inport  Port=11  OutDataTypeStr=Bus:CAN_FD_MESSAGE_BUS
  CCAN_ADCU_GW_Body_0x321FromInData : Inport  Port=12  OutDataTypeStr=Bus:CAN_FD_MESSAGE_BUS
  CCAN_ADCU_GW_DMS_0x4A0FromInData : Inport  Port=13  OutDataTypeStr=Bus:CAN_FD_MESSAGE_BUS
  CCAN_ADCU_GW_EMS_Engstatus_0x142FromInData : Inport  Port=14  OutDataTypeStr=Bus:CAN_FD_MESSAGE_BUS
  CCAN_ADCU_GW_EMS_Sts_0x151FromInData : Inport  Port=15  OutDataTypeStr=Bus:CAN_FD_MESSAGE_BUS
  CCAN_ADCU_GW_EMS_TqWhl_0x111FromInData : Inport  Port=16  OutDataTypeStr=Bus:CAN_FD_MESSAGE_BUS
  CCAN_ADCU_GW_EMS_Tq_0x101FromInData : Inport  Port=17  OutDataTypeStr=Bus:CAN_FD_MESSAGE_BUS
  CCAN_ADCU_GW_EMS_WhlTq_0x107FromInData : Inport  Port=18  OutDataTypeStr=Bus:CAN_FD_MESSAGE_BUS
  CCAN_ADCU_GW_IC_0x510FromInData : Inport  Port=19  OutDataTypeStr=Bus:CAN_FD_MESSAGE_BUS
  CCAN_ADCU_GW_IC_Time_0x581FromInData : Inport  Port=20  OutDataTypeStr=Bus:CAN_FD_MESSAGE_BUS
  CCAN_ADCU_GW_MP5_0x530FromInData : Inport  Port=21  OutDataTypeStr=Bus:CAN_FD_MESSAGE_BUS
  CCAN_ADCU_GW_MP5_AVM_0x3A1FromInData : Inport  Port=22  OutDataTypeStr=Bus:CAN_FD_MESSAGE_BUS
  CCAN_ADCU_GW_MP5_LicensePlateNum_0x375FromInData : Inport  Port=23  OutDataTypeStr=Bus:CAN_FD_MESSAGE_BUS
  CCAN_ADCU_GW_MP5_NAV_0x533FromInData : Inport  Port=24  OutDataTypeStr=Bus:CAN_FD_MESSAGE_BUS
  CCAN_ADCU_GW_SRS_0x350FromInData : Inport  Port=25  OutDataTypeStr=Bus:CAN_FD_MESSAGE_BUS
  CCAN_ADCU_GW_TCU_GearInfo_0x123FromInData : Inport  Port=26  OutDataTypeStr=Bus:CAN_FD_MESSAGE_BUS
  CCAN_ADCU_SAS_Sensor_0x175FromInData : Inport  Port=27  OutDataTypeStr=Bus:CAN_FD_MESSAGE_BUS
  CCAN_ADCU_SRR_FL_0x27BFromInData : Inport  Port=28  OutDataTypeStr=Bus:CAN_FD_MESSAGE_BUS
  CCAN_ADCU_SWM_Body_0x31AFromInData : Inport  Port=29  OutDataTypeStr=Bus:CAN_FD_MESSAGE_BUS
  CCAN_ADCU_SWM_MRR_0x31BFromInData : Inport  Port=30  OutDataTypeStr=Bus:CAN_FD_MESSAGE_BUS
  CCAN_ADCU_Tester_DiagFuncReqFromInData : Inport  Port=31  OutDataTypeStr=Bus:CAN_FD_MESSAGE_BUS
  CCAN_ADCU_Tester_DiagReqToADCUFromInData : Inport  Port=32  OutDataTypeStr=Bus:CAN_FD_MESSAGE_BUS
  CCAN_ADCU_ABS_Sts_0x221 : Subsystem  TreatAsAtomicUnit=on
  CCAN_ADCU_BSD_0x275 : Subsystem  TreatAsAtomicUnit=on
  CCAN_ADCU_EPS_Advanced_0x176 : Subsystem  TreatAsAtomicUnit=on
  CCAN_ADCU_ESP_Advanced_0x234 : Subsystem  TreatAsAtomicUnit=on
  CCAN_ADCU_ESP_AxAy_0x242 : Subsystem  TreatAsAtomicUnit=on
  CCAN_ADCU_ESP_Direction_0x235 : Subsystem  TreatAsAtomicUnit=on
  CCAN_ADCU_ESP_Pressure_0x241 : Subsystem  TreatAsAtomicUnit=on
  CCAN_ADCU_ESP_RAW_0x212 : Subsystem  TreatAsAtomicUnit=on
  CCAN_ADCU_ESP_Status_0x243 : Subsystem  TreatAsAtomicUnit=on
  CCAN_ADCU_GW_AWD_0x251 : Subsystem  TreatAsAtomicUnit=on
  CCAN_ADCU_GW_BCM_Door_0x310 : Subsystem  TreatAsAtomicUnit=on
  CCAN_ADCU_GW_Body_0x321 : Subsystem  TreatAsAtomicUnit=on
  CCAN_ADCU_GW_DMS_0x4A0 : Subsystem  TreatAsAtomicUnit=on
  CCAN_ADCU_GW_EMS_Engstatus_0x142 : Subsystem  TreatAsAtomicUnit=on
  CCAN_ADCU_GW_EMS_Sts_0x151 : Subsystem  TreatAsAtomicUnit=on
  CCAN_ADCU_GW_EMS_TqWhl_0x111 : Subsystem  TreatAsAtomicUnit=on
  CCAN_ADCU_GW_EMS_Tq_0x101 : Subsystem  TreatAsAtomicUnit=on
  CCAN_ADCU_GW_EMS_WhlTq_0x107 : Subsystem  TreatAsAtomicUnit=on
  CCAN_ADCU_GW_IC_0x510 : Subsystem  TreatAsAtomicUnit=on
  CCAN_ADCU_GW_IC_Time_0x581 : Subsystem  TreatAsAtomicUnit=on
  CCAN_ADCU_GW_MP5_0x530 : Subsystem  TreatAsAtomicUnit=on
  CCAN_ADCU_GW_MP5_AVM_0x3A1 : Subsystem  TreatAsAtomicUnit=on
  CCAN_ADCU_GW_MP5_LicensePlateNum_0x375 : Subsystem  TreatAsAtomicUnit=on
  CCAN_ADCU_GW_MP5_NAV_0x533 : Subsystem  TreatAsAtomicUnit=on
  CCAN_ADCU_GW_SRS_0x350 : Subsystem  TreatAsAtomicUnit=on
  CCAN_ADCU_GW_TCU_GearInfo_0x123 : Subsystem  TreatAsAtomicUnit=on
  CCAN_ADCU_SAS_Sensor_0x175 : Subsystem  TreatAsAtomicUnit=on
  CCAN_ADCU_SRR_FL_0x27B : Subsystem  TreatAsAtomicUnit=on
  CCAN_ADCU_SWM_Body_0x31A : Subsystem  TreatAsAtomicUnit=on
  CCAN_ADCU_SWM_MRR_0x31B : Subsystem  TreatAsAtomicUnit=on
  CCAN_ADCU_Tester_DiagFuncReq : Subsystem  TreatAsAtomicUnit=on
  CCAN_ADCU_Tester_DiagReqToADCU : Subsystem  TreatAsAtomicUnit=on
  CCAN_ADCU_ABS_Sts_0x221FromOutData : Outport  OutDataTypeStr=Bus:CCAN_ADCU_ABS_Sts_0x221
  CCAN_ADCU_BSD_0x275FromOutData : Outport  Port=2  OutDataTypeStr=Bus:CCAN_ADCU_BSD_0x275
  CCAN_ADCU_EPS_Advanced_0x176FromOutData : Outport  Port=3  OutDataTypeStr=Bus:CCAN_ADCU_EPS_Advanced_0x176
  CCAN_ADCU_ESP_Advanced_0x234FromOutData : Outport  Port=4  OutDataTypeStr=Bus:CCAN_ADCU_ESP_Advanced_0x234
  CCAN_ADCU_ESP_AxAy_0x242FromOutData : Outport  Port=5  OutDataTypeStr=Bus:CCAN_ADCU_ESP_AxAy_0x242
  CCAN_ADCU_ESP_Direction_0x235FromOutData : Outport  Port=6  OutDataTypeStr=Bus:CCAN_ADCU_ESP_Direction_0x235
  CCAN_ADCU_ESP_Pressure_0x241FromOutData : Outport  Port=7  OutDataTypeStr=Bus:CCAN_ADCU_ESP_Pressure_0x241
  CCAN_ADCU_ESP_RAW_0x212FromOutData : Outport  Port=8  OutDataTypeStr=Bus:CCAN_ADCU_ESP_RAW_0x212
  CCAN_ADCU_ESP_Status_0x243FromOutData : Outport  Port=9  OutDataTypeStr=Bus:CCAN_ADCU_ESP_Status_0x243
  CCAN_ADCU_GW_AWD_0x251FromOutData : Outport  Port=10  OutDataTypeStr=Bus:CCAN_ADCU_GW_AWD_0x251
  CCAN_ADCU_GW_BCM_Door_0x310FromOutData : Outport  Port=11  OutDataTypeStr=Bus:CCAN_ADCU_GW_BCM_Door_0x310
  CCAN_ADCU_GW_Body_0x321FromOutData : Outport  Port=12  OutDataTypeStr=Bus:CCAN_ADCU_GW_Body_0x321
  CCAN_ADCU_GW_DMS_0x4A0FromOutData : Outport  Port=13  OutDataTypeStr=Bus:CCAN_ADCU_GW_DMS_0x4A0
  CCAN_ADCU_GW_EMS_Engstatus_0x142FromOutData : Outport  Port=14  OutDataTypeStr=Bus:CCAN_ADCU_GW_EMS_Engstatus_0x142
  CCAN_ADCU_GW_EMS_Sts_0x151FromOutData : Outport  Port=15  OutDataTypeStr=Bus:CCAN_ADCU_GW_EMS_Sts_0x151
  CCAN_ADCU_GW_EMS_TqWhl_0x111FromOutData : Outport  Port=16  OutDataTypeStr=Bus:CCAN_ADCU_GW_EMS_TqWhl_0x111
  CCAN_ADCU_GW_EMS_Tq_0x101FromOutData : Outport  Port=17  OutDataTypeStr=Bus:CCAN_ADCU_GW_EMS_Tq_0x101
  CCAN_ADCU_GW_EMS_WhlTq_0x107FromOutData : Outport  Port=18  OutDataTypeStr=Bus:CCAN_ADCU_GW_EMS_WhlTq_0x107
  CCAN_ADCU_GW_IC_0x510FromOutData : Outport  Port=19  OutDataTypeStr=Bus:CCAN_ADCU_GW_IC_0x510
  CCAN_ADCU_GW_IC_Time_0x581FromOutData : Outport  Port=20  OutDataTypeStr=Bus:CCAN_ADCU_GW_IC_Time_0x581
  CCAN_ADCU_GW_MP5_0x530FromOutData : Outport  Port=21  OutDataTypeStr=Bus:CCAN_ADCU_GW_MP5_0x530
  CCAN_ADCU_GW_MP5_AVM_0x3A1FromOutData : Outport  Port=22  OutDataTypeStr=Bus:CCAN_ADCU_GW_MP5_AVM_0x3A1
  CCAN_ADCU_GW_MP5_LicensePlateNum_0x375FromOutData : Outport  Port=23  OutDataTypeStr=Bus:CCAN_ADCU_GW_MP5_LicensePlateNum_0x375
  CCAN_ADCU_GW_MP5_NAV_0x533FromOutData : Outport  Port=24  OutDataTypeStr=Bus:CCAN_ADCU_GW_MP5_NAV_0x533
  CCAN_ADCU_GW_SRS_0x350FromOutData : Outport  Port=25  OutDataTypeStr=Bus:CCAN_ADCU_GW_SRS_0x350
  CCAN_ADCU_GW_TCU_GearInfo_0x123FromOutData : Outport  Port=26  OutDataTypeStr=Bus:CCAN_ADCU_GW_TCU_GearInfo_0x123
  CCAN_ADCU_SAS_Sensor_0x175FromOutData : Outport  Port=27  OutDataTypeStr=Bus:CCAN_ADCU_SAS_Sensor_0x175
  CCAN_ADCU_SRR_FL_0x27BFromOutData : Outport  Port=28  OutDataTypeStr=Bus:CCAN_ADCU_SRR_FL_0x27B
  CCAN_ADCU_SWM_Body_0x31AFromOutData : Outport  Port=29  OutDataTypeStr=Bus:CCAN_ADCU_SWM_Body_0x31A
  CCAN_ADCU_SWM_MRR_0x31BFromOutData : Outport  Port=30  OutDataTypeStr=Bus:CCAN_ADCU_SWM_MRR_0x31B
  CCAN_ADCU_Tester_DiagFuncReqFromOutData : Outport  Port=31  OutDataTypeStr=Bus:CCAN_ADCU_Tester_DiagFuncReq
  CCAN_ADCU_Tester_DiagReqToADCUFromOutData : Outport  Port=32  OutDataTypeStr=Bus:CCAN_ADCU_Tester_DiagReqToADCU
  wires:
  CCAN_ADCU_ABS_Sts_0x221/1(CCAN_ADCU_ABS_Sts_0x221FromOutData) -> CCAN_ADCU_ABS_Sts_0x221FromOutData/1  "CCAN_ADCU_ABS_Sts_0x221FromOutData"
  CCAN_ADCU_ABS_Sts_0x221FromInData/1 -> CCAN_ADCU_ABS_Sts_0x221/1(CCAN_ADCU_ABS_Sts_0x221FromInData)  "CCAN_ADCU_ABS_Sts_0x221FromInData"
  CCAN_ADCU_BSD_0x275/1(CCAN_ADCU_BSD_0x275FromOutData) -> CCAN_ADCU_BSD_0x275FromOutData/1  "CCAN_ADCU_BSD_0x275FromOutData"
  CCAN_ADCU_BSD_0x275FromInData/1 -> CCAN_ADCU_BSD_0x275/1(CCAN_ADCU_BSD_0x275FromInData)  "CCAN_ADCU_BSD_0x275FromInData"
  CCAN_ADCU_EPS_Advanced_0x176/1(CCAN_ADCU_EPS_Advanced_0x176FromOutData) -> CCAN_ADCU_EPS_Advanced_0x176FromOutData/1  "CCAN_ADCU_EPS_Advanced_0x176FromOutData"
  CCAN_ADCU_EPS_Advanced_0x176FromInData/1 -> CCAN_ADCU_EPS_Advanced_0x176/1(CCAN_ADCU_EPS_Advanced_0x176FromInData)  "CCAN_ADCU_EPS_Advanced_0x176FromInData"
  CCAN_ADCU_ESP_Advanced_0x234/1(CCAN_ADCU_ESP_Advanced_0x234FromOutData) -> CCAN_ADCU_ESP_Advanced_0x234FromOutData/1  "CCAN_ADCU_ESP_Advanced_0x234FromOutData"
  CCAN_ADCU_ESP_Advanced_0x234FromInData/1 -> CCAN_ADCU_ESP_Advanced_0x234/1(CCAN_ADCU_ESP_Advanced_0x234FromInData)  "CCAN_ADCU_ESP_Advanced_0x234FromInData"
  CCAN_ADCU_ESP_AxAy_0x242/1(CCAN_ADCU_ESP_AxAy_0x242FromOutData) -> CCAN_ADCU_ESP_AxAy_0x242FromOutData/1  "CCAN_ADCU_ESP_AxAy_0x242FromOutData"
  CCAN_ADCU_ESP_AxAy_0x242FromInData/1 -> CCAN_ADCU_ESP_AxAy_0x242/1(CCAN_ADCU_ESP_AxAy_0x242FromInData)  "CCAN_ADCU_ESP_AxAy_0x242FromInData"
  CCAN_ADCU_ESP_Direction_0x235/1(CCAN_ADCU_ESP_Direction_0x235FromOutData) -> CCAN_ADCU_ESP_Direction_0x235FromOutData/1  "CCAN_ADCU_ESP_Direction_0x235FromOutData"
  CCAN_ADCU_ESP_Direction_0x235FromInData/1 -> CCAN_ADCU_ESP_Direction_0x235/1(CCAN_ADCU_ESP_Direction_0x235FromInData)  "CCAN_ADCU_ESP_Direction_0x235FromInData"
  CCAN_ADCU_ESP_Pressure_0x241/1(CCAN_ADCU_ESP_Pressure_0x241FromOutData) -> CCAN_ADCU_ESP_Pressure_0x241FromOutData/1  "CCAN_ADCU_ESP_Pressure_0x241FromOutData"
  CCAN_ADCU_ESP_Pressure_0x241FromInData/1 -> CCAN_ADCU_ESP_Pressure_0x241/1(CCAN_ADCU_ESP_Pressure_0x241FromInData)  "CCAN_ADCU_ESP_Pressure_0x241FromInData"
  CCAN_ADCU_ESP_RAW_0x212/1(CCAN_ADCU_ESP_RAW_0x212FromOutData) -> CCAN_ADCU_ESP_RAW_0x212FromOutData/1  "CCAN_ADCU_ESP_RAW_0x212FromOutData"
  CCAN_ADCU_ESP_RAW_0x212FromInData/1 -> CCAN_ADCU_ESP_RAW_0x212/1(CCAN_ADCU_ESP_RAW_0x212FromInData)  "CCAN_ADCU_ESP_RAW_0x212FromInData"
  CCAN_ADCU_ESP_Status_0x243/1(CCAN_ADCU_ESP_Status_0x243FromOutData) -> CCAN_ADCU_ESP_Status_0x243FromOutData/1  "CCAN_ADCU_ESP_Status_0x243FromOutData"
  CCAN_ADCU_ESP_Status_0x243FromInData/1 -> CCAN_ADCU_ESP_Status_0x243/1(CCAN_ADCU_ESP_Status_0x243FromInData)  "CCAN_ADCU_ESP_Status_0x243FromInData"
  CCAN_ADCU_GW_AWD_0x251/1(CCAN_ADCU_GW_AWD_0x251FromOutData) -> CCAN_ADCU_GW_AWD_0x251FromOutData/1  "CCAN_ADCU_GW_AWD_0x251FromOutData"
  CCAN_ADCU_GW_AWD_0x251FromInData/1 -> CCAN_ADCU_GW_AWD_0x251/1(CCAN_ADCU_GW_AWD_0x251FromInData)  "CCAN_ADCU_GW_AWD_0x251FromInData"
  CCAN_ADCU_GW_BCM_Door_0x310/1(CCAN_ADCU_GW_BCM_Door_0x310FromOutData) -> CCAN_ADCU_GW_BCM_Door_0x310FromOutData/1  "CCAN_ADCU_GW_BCM_Door_0x310FromOutData"
  CCAN_ADCU_GW_BCM_Door_0x310FromInData/1 -> CCAN_ADCU_GW_BCM_Door_0x310/1(CCAN_ADCU_GW_BCM_Door_0x310FromInData)  "CCAN_ADCU_GW_BCM_Door_0x310FromInData"
  CCAN_ADCU_GW_Body_0x321/1(CCAN_ADCU_GW_Body_0x321FromOutData) -> CCAN_ADCU_GW_Body_0x321FromOutData/1  "CCAN_ADCU_GW_Body_0x321FromOutData"
  CCAN_ADCU_GW_Body_0x321FromInData/1 -> CCAN_ADCU_GW_Body_0x321/1(CCAN_ADCU_GW_Body_0x321FromInData)  "CCAN_ADCU_GW_Body_0x321FromInData"
  CCAN_ADCU_GW_DMS_0x4A0/1(CCAN_ADCU_GW_DMS_0x4A0FromOutData) -> CCAN_ADCU_GW_DMS_0x4A0FromOutData/1  "CCAN_ADCU_GW_DMS_0x4A0FromOutData"
  CCAN_ADCU_GW_DMS_0x4A0FromInData/1 -> CCAN_ADCU_GW_DMS_0x4A0/1(CCAN_ADCU_GW_DMS_0x4A0FromInData)  "CCAN_ADCU_GW_DMS_0x4A0FromInData"
  CCAN_ADCU_GW_EMS_Engstatus_0x142/1(CCAN_ADCU_GW_EMS_Engstatus_0x142FromOutData) -> CCAN_ADCU_GW_EMS_Engstatus_0x142FromOutData/1  "CCAN_ADCU_GW_EMS_Engstatus_0x142FromOutData"
  CCAN_ADCU_GW_EMS_Engstatus_0x142FromInData/1 -> CCAN_ADCU_GW_EMS_Engstatus_0x142/1(CCAN_ADCU_GW_EMS_Engstatus_0x142FromInData)  "CCAN_ADCU_GW_EMS_Engstatus_0x142FromInData"
  CCAN_ADCU_GW_EMS_Sts_0x151/1(CCAN_ADCU_GW_EMS_Sts_0x151FromOutData) -> CCAN_ADCU_GW_EMS_Sts_0x151FromOutData/1  "CCAN_ADCU_GW_EMS_Sts_0x151FromOutData"
  CCAN_ADCU_GW_EMS_Sts_0x151FromInData/1 -> CCAN_ADCU_GW_EMS_Sts_0x151/1(CCAN_ADCU_GW_EMS_Sts_0x151FromInData)  "CCAN_ADCU_GW_EMS_Sts_0x151FromInData"
  CCAN_ADCU_GW_EMS_TqWhl_0x111/1(CCAN_ADCU_GW_EMS_TqWhl_0x111FromOutData) -> CCAN_ADCU_GW_EMS_TqWhl_0x111FromOutData/1  "CCAN_ADCU_GW_EMS_TqWhl_0x111FromOutData"
  CCAN_ADCU_GW_EMS_TqWhl_0x111FromInData/1 -> CCAN_ADCU_GW_EMS_TqWhl_0x111/1(CCAN_ADCU_GW_EMS_TqWhl_0x111FromInData)  "CCAN_ADCU_GW_EMS_TqWhl_0x111FromInData"
  CCAN_ADCU_GW_EMS_Tq_0x101/1(CCAN_ADCU_GW_EMS_Tq_0x101FromOutData) -> CCAN_ADCU_GW_EMS_Tq_0x101FromOutData/1  "CCAN_ADCU_GW_EMS_Tq_0x101FromOutData"
  CCAN_ADCU_GW_EMS_Tq_0x101FromInData/1 -> CCAN_ADCU_GW_EMS_Tq_0x101/1(CCAN_ADCU_GW_EMS_Tq_0x101FromInData)  "CCAN_ADCU_GW_EMS_Tq_0x101FromInData"
  CCAN_ADCU_GW_EMS_WhlTq_0x107/1(CCAN_ADCU_GW_EMS_WhlTq_0x107FromOutData) -> CCAN_ADCU_GW_EMS_WhlTq_0x107FromOutData/1  "CCAN_ADCU_GW_EMS_WhlTq_0x107FromOutData"
  CCAN_ADCU_GW_EMS_WhlTq_0x107FromInData/1 -> CCAN_ADCU_GW_EMS_WhlTq_0x107/1(CCAN_ADCU_GW_EMS_WhlTq_0x107FromInData)  "CCAN_ADCU_GW_EMS_WhlTq_0x107FromInData"
  CCAN_ADCU_GW_IC_0x510/1(CCAN_ADCU_GW_IC_0x510FromOutData) -> CCAN_ADCU_GW_IC_0x510FromOutData/1  "CCAN_ADCU_GW_IC_0x510FromOutData"
  CCAN_ADCU_GW_IC_0x510FromInData/1 -> CCAN_ADCU_GW_IC_0x510/1(CCAN_ADCU_GW_IC_0x510FromInData)  "CCAN_ADCU_GW_IC_0x510FromInData"
  CCAN_ADCU_GW_IC_Time_0x581/1(CCAN_ADCU_GW_IC_Time_0x581FromOutData) -> CCAN_ADCU_GW_IC_Time_0x581FromOutData/1  "CCAN_ADCU_GW_IC_Time_0x581FromOutData"
  CCAN_ADCU_GW_IC_Time_0x581FromInData/1 -> CCAN_ADCU_GW_IC_Time_0x581/1(CCAN_ADCU_GW_IC_Time_0x581FromInData)  "CCAN_ADCU_GW_IC_Time_0x581FromInData"
  CCAN_ADCU_GW_MP5_0x530/1(CCAN_ADCU_GW_MP5_0x530FromOutData) -> CCAN_ADCU_GW_MP5_0x530FromOutData/1  "CCAN_ADCU_GW_MP5_0x530FromOutData"
  CCAN_ADCU_GW_MP5_0x530FromInData/1 -> CCAN_ADCU_GW_MP5_0x530/1(CCAN_ADCU_GW_MP5_0x530FromInData)  "CCAN_ADCU_GW_MP5_0x530FromInData"
  CCAN_ADCU_GW_MP5_AVM_0x3A1/1(CCAN_ADCU_GW_MP5_AVM_0x3A1FromOutData) -> CCAN_ADCU_GW_MP5_AVM_0x3A1FromOutData/1  "CCAN_ADCU_GW_MP5_AVM_0x3A1FromOutData"
  CCAN_ADCU_GW_MP5_AVM_0x3A1FromInData/1 -> CCAN_ADCU_GW_MP5_AVM_0x3A1/1(CCAN_ADCU_GW_MP5_AVM_0x3A1FromInData)  "CCAN_ADCU_GW_MP5_AVM_0x3A1FromInData"
  CCAN_ADCU_GW_MP5_LicensePlateNum_0x375/1(CCAN_ADCU_GW_MP5_LicensePlateNum_0x375FromOutData) -> CCAN_ADCU_GW_MP5_LicensePlateNum_0x375FromOutData/1  "CCAN_ADCU_GW_MP5_LicensePlateNum_0x375FromOutData"
  CCAN_ADCU_GW_MP5_LicensePlateNum_0x375FromInData/1 -> CCAN_ADCU_GW_MP5_LicensePlateNum_0x375/1(CCAN_ADCU_GW_MP5_LicensePlateNum_0x375FromInData)  "CCAN_ADCU_GW_MP5_LicensePlateNum_0x375FromInData"
  CCAN_ADCU_GW_MP5_NAV_0x533/1(CCAN_ADCU_GW_MP5_NAV_0x533FromOutData) -> CCAN_ADCU_GW_MP5_NAV_0x533FromOutData/1  "CCAN_ADCU_GW_MP5_NAV_0x533FromOutData"
  CCAN_ADCU_GW_MP5_NAV_0x533FromInData/1 -> CCAN_ADCU_GW_MP5_NAV_0x533/1(CCAN_ADCU_GW_MP5_NAV_0x533FromInData)  "CCAN_ADCU_GW_MP5_NAV_0x533FromInData"
  CCAN_ADCU_GW_SRS_0x350/1(CCAN_ADCU_GW_SRS_0x350FromOutData) -> CCAN_ADCU_GW_SRS_0x350FromOutData/1  "CCAN_ADCU_GW_SRS_0x350FromOutData"
  CCAN_ADCU_GW_SRS_0x350FromInData/1 -> CCAN_ADCU_GW_SRS_0x350/1(CCAN_ADCU_GW_SRS_0x350FromInData)  "CCAN_ADCU_GW_SRS_0x350FromInData"
  CCAN_ADCU_GW_TCU_GearInfo_0x123/1(CCAN_ADCU_GW_TCU_GearInfo_0x123FromOutData) -> CCAN_ADCU_GW_TCU_GearInfo_0x123FromOutData/1  "CCAN_ADCU_GW_TCU_GearInfo_0x123FromOutData"
  CCAN_ADCU_GW_TCU_GearInfo_0x123FromInData/1 -> CCAN_ADCU_GW_TCU_GearInfo_0x123/1(CCAN_ADCU_GW_TCU_GearInfo_0x123FromInData)  "CCAN_ADCU_GW_TCU_GearInfo_0x123FromInData"
  CCAN_ADCU_SAS_Sensor_0x175/1(CCAN_ADCU_SAS_Sensor_0x175FromOutData) -> CCAN_ADCU_SAS_Sensor_0x175FromOutData/1  "CCAN_ADCU_SAS_Sensor_0x175FromOutData"
  CCAN_ADCU_SAS_Sensor_0x175FromInData/1 -> CCAN_ADCU_SAS_Sensor_0x175/1(CCAN_ADCU_SAS_Sensor_0x175FromInData)  "CCAN_ADCU_SAS_Sensor_0x175FromInData"
  CCAN_ADCU_SRR_FL_0x27B/1(CCAN_ADCU_SRR_FL_0x27BFromOutData) -> CCAN_ADCU_SRR_FL_0x27BFromOutData/1  "CCAN_ADCU_SRR_FL_0x27BFromOutData"
  CCAN_ADCU_SRR_FL_0x27BFromInData/1 -> CCAN_ADCU_SRR_FL_0x27B/1(CCAN_ADCU_SRR_FL_0x27BFromInData)  "CCAN_ADCU_SRR_FL_0x27BFromInData"
  CCAN_ADCU_SWM_Body_0x31A/1(CCAN_ADCU_SWM_Body_0x31AFromOutData) -> CCAN_ADCU_SWM_Body_0x31AFromOutData/1  "CCAN_ADCU_SWM_Body_0x31AFromOutData"
  CCAN_ADCU_SWM_Body_0x31AFromInData/1 -> CCAN_ADCU_SWM_Body_0x31A/1(CCAN_ADCU_SWM_Body_0x31AFromInData)  "CCAN_ADCU_SWM_Body_0x31AFromInData"
  CCAN_ADCU_SWM_MRR_0x31B/1(CCAN_ADCU_SWM_MRR_0x31BFromOutData) -> CCAN_ADCU_SWM_MRR_0x31BFromOutData/1  "CCAN_ADCU_SWM_MRR_0x31BFromOutData"
  CCAN_ADCU_SWM_MRR_0x31BFromInData/1 -> CCAN_ADCU_SWM_MRR_0x31B/1(CCAN_ADCU_SWM_MRR_0x31BFromInData)  "CCAN_ADCU_SWM_MRR_0x31BFromInData"
  CCAN_ADCU_Tester_DiagFuncReq/1(CCAN_ADCU_Tester_DiagFuncReqFromOutData) -> CCAN_ADCU_Tester_DiagFuncReqFromOutData/1  "CCAN_ADCU_Tester_DiagFuncReqFromOutData"
  CCAN_ADCU_Tester_DiagFuncReqFromInData/1 -> CCAN_ADCU_Tester_DiagFuncReq/1(CCAN_ADCU_Tester_DiagFuncReqFromInData)  "CCAN_ADCU_Tester_DiagFuncReqFromInData"
  CCAN_ADCU_Tester_DiagReqToADCU/1(CCAN_ADCU_Tester_DiagReqToADCUFromOutData) -> CCAN_ADCU_Tester_DiagReqToADCUFromOutData/1  "CCAN_ADCU_Tester_DiagReqToADCUFromOutData"
  CCAN_ADCU_Tester_DiagReqToADCUFromInData/1 -> CCAN_ADCU_Tester_DiagReqToADCU/1(CCAN_ADCU_Tester_DiagReqToADCUFromInData)  "CCAN_ADCU_Tester_DiagReqToADCUFromInData"
